simulink model "sim3"  (R2023a)
settings: Solver=VariableStepAuto  StartTime=0  StopTime=1.6  RelTol=1e-8
settings Model: Creator=vasil  LastModifiedBy=vasil

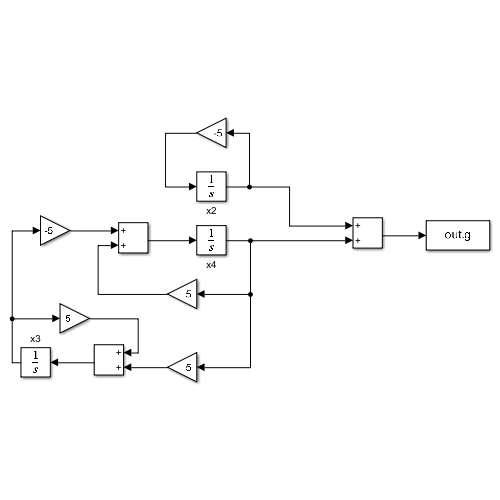
[thumbnail: Simulink's stored preview of the top-level diagram]
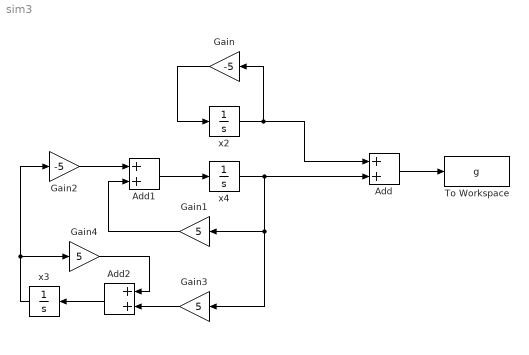
== system sim3 ==
  Add : Sum
  Add1 : Sum
  Add2 : Sum
  Gain : Gain  Gain=-5
  Gain1 : Gain  Gain=5
  Gain2 : Gain  Gain=-5
  Gain3 : Gain  Gain=5
  Gain4 : Gain  Gain=5
  To Workspace : ToWorkspace  VariableName=g  SaveFormat=Timeseries  SampleTime=-1
  x2 : Integrator
  x3 : Integrator
  x4 : Integrator  InitialCondition=1
  wires:
  Add/1 -> To Workspace/1
  x2/1 -> Gain/1, Add/1
  x4/1 -> Gain1/1, Gain3/1, Add/2
  Add1/1 -> x4/1
  Gain/1 -> x2/1
  Gain1/1 -> Add1/2
  Gain2/1 -> Add1/1
  Add2/1 -> x3/1
  x3/1 -> Gain4/1, Gain2/1
  Gain3/1 -> Add2/2
  Gain4/1 -> Add2/1
